simulink model "Quaternion_from_NodeMCU"  (R2018b)
settings: Solver=VariableStepAuto  StartTime=0.0  StopTime=inf  FixedStep=0.01  RelTol=1e-3
undefined symbols (not defined in the file): LF, serial
libraries: instrumentlib x4, sm_lib x4, nesl_utility x4, sharedtransform x1
settings Model: Creator=gelli  LastModifiedBy=gelli

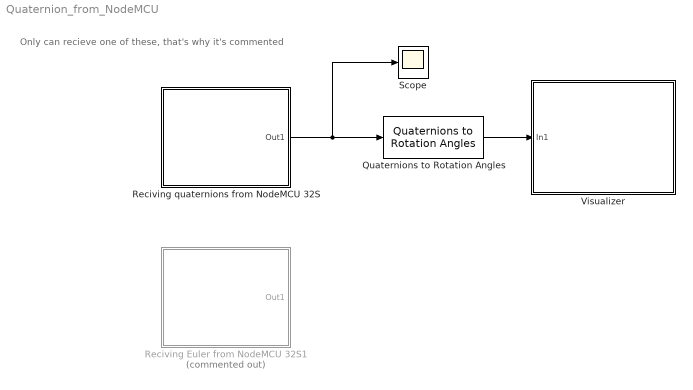
== system Quaternion_from_NodeMCU ==
  note: Only can recieve one of these, that's why it's commented
  Quaternions to Rotation Angles : sharedtransform/Quaternions to Rotation Angles  rotationOrder=XYZ  aMode=aMode
      settings: SourceProductBaseCode=AE
  Reciving Euler from NodeMCU 32S1 : Subsystem  Commented=on
      mask Display: image('Picture_of_NodeMCU.jpg');
  Reciving quaternions from NodeMCU 32S : Subsystem
      mask Display: image('Picture_of_NodeMCU.jpg');
  Scope : Scope
  Visualizer : Subsystem
  wires:
  Reciving quaternions from NodeMCU 32S/1(Out1) -> Quaternions to Rotation Angles/1, Scope/1
  Quaternions to Rotation Angles/1 -> Visualizer/1(In1)

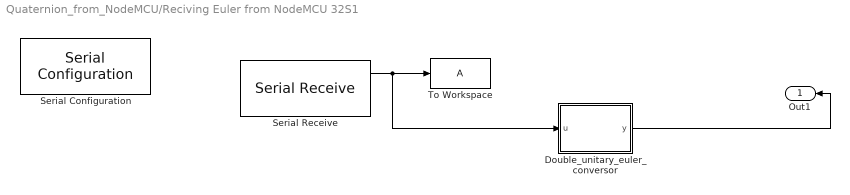
== system Quaternion_from_NodeMCU/Reciving Euler from NodeMCU 32S1 ==
  Double_unitary_euler_conversor : MATLAB Function  TreatAsAtomicUnit=on
  Serial Configuration : instrumentlib/Serial Configuration  Priority=-200000  ComPortMenu=COM6  ComPort=COM6  ObjConstructor=serial('COM6');  BaudRate=115200  DataBits=8  Parity=none  StopBits=1  FlowControl=none  Timeout=10  ByteOrder=LittleEndian
  Serial Receive : instrumentlib/Serial Receive  ComPortMenu=COM6  ComPort=COM6  ObjConstructor=serial('COM6');  Header=R  Terminator=LF ('\n')  DataSize=3  DataType=uint8  EnableBlockingMode=off  ActionDataUnavailable=Output last received value  CustomValue=0  SampleTime=0.001
  To Workspace : ToWorkspace  VariableName=A  SaveFormat=Timeseries  SampleTime=-1
  Out1 : Outport
  wires:
  Double_unitary_euler_conversor/1(y) -> Out1/1
  Serial Receive/1 -> Double_unitary_euler_conversor/1(u), To Workspace/1

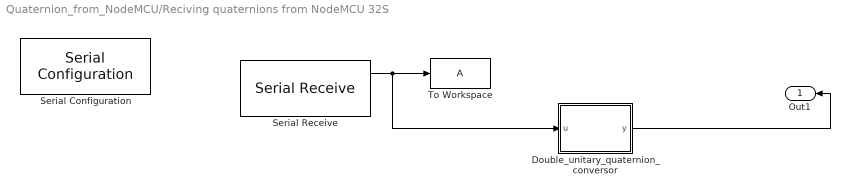
== system Quaternion_from_NodeMCU/Reciving quaternions from NodeMCU 32S ==
  Double_unitary_quaternion_conversor : MATLAB Function  TreatAsAtomicUnit=on
  Serial Configuration : instrumentlib/Serial Configuration  Priority=-200000  ComPortMenu=COM6  ComPort=COM6  ObjConstructor=serial('COM6');  BaudRate=115200  DataBits=8  Parity=none  StopBits=1  FlowControl=none  Timeout=10  ByteOrder=LittleEndian
  Serial Receive : instrumentlib/Serial Receive  ComPortMenu=COM6  ComPort=COM6  ObjConstructor=serial('COM6');  Header=R  Terminator=LF ('\n')  DataSize=4  DataType=uint8  EnableBlockingMode=off  ActionDataUnavailable=Output last received value  CustomValue=0  SampleTime=0.01
  To Workspace : ToWorkspace  VariableName=A  SaveFormat=Timeseries  SampleTime=-1
  Out1 : Outport
  wires:
  Double_unitary_quaternion_conversor/1(y) -> Out1/1
  Serial Receive/1 -> Double_unitary_quaternion_conversor/1(u), To Workspace/1

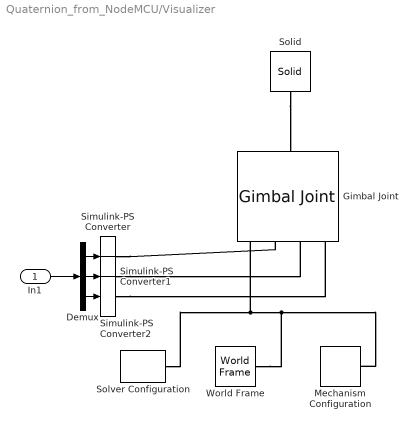
== system Quaternion_from_NodeMCU/Visualizer ==
  In1 : Inport
  Demux : Demux  Outputs=3
  Gimbal Joint : sm_lib/Joints/Gimbal Joint  SenseConstraintForce=off  SenseConstraintForceX=off  SenseConstraintForceY=off  SenseConstraintForceZ=off  SenseConstraintTorque=off  SenseConstraintTorqueX=off  SenseConstraintTorqueY=off  SenseConstraintTorqueZ=off  SenseTotalForce=off  SenseTotalForceX=off  SenseTotalForceY=off  SenseTotalForceZ=off  SenseTotalTorque=off  SenseTotalTorqueX=off  SenseTotalTorqueY=off  SenseTotalTorqueZ=off  CompositeWrenchDir=FollowerOnBase  CompositeWrenchFrame=BaseFrame  RxEquilibriumPosition=0  RxEquilibriumPositionUnits=deg  RxSpringStiffness=0  RxSpringStiffnessUnits=N*m/deg  RxDampingCoefficient=0  RxDampingCoefficientUnits=N*m/(deg/s)  RxTorqueActuationMode=ComputedTorque  RxMotionActuationMode=InputMotion  RxSensePosition=off  RxSenseVelocity=off  RxSenseAcceleration=off  RxSenseTorqueForce=off  RxPositionTargetSpecify=off  RxPositionTargetPriority=High  RxPositionTargetValue=0  RxPositionTargetValueUnits=deg  RxVelocityTargetSpecify=off  RxVelocityTargetPriority=High  RxVelocityTargetValue=0  RxVelocityTargetValueUnits=deg/s  RyEquilibriumPosition=0  RyEquilibriumPositionUnits=deg  RySpringStiffness=0  RySpringStiffnessUnits=N*m/deg  RyDampingCoefficient=0  RyDampingCoefficientUnits=N*m/(deg/s)  RyTorqueActuationMode=ComputedTorque  RyMotionActuationMode=InputMotion  RySensePosition=off  RySenseVelocity=off  RySenseAcceleration=off  RySenseTorqueForce=off  RyPositionTargetSpecify=off  RyPositionTargetPriority=High  RyPositionTargetValue=0  RyPositionTargetValueUnits=deg  RyVelocityTargetSpecify=off  RyVelocityTargetPriority=High  RyVelocityTargetValue=0  RyVelocityTargetValueUnits=deg/s  RzEquilibriumPosition=0  RzEquilibriumPositionUnits=deg  RzSpringStiffness=0  RzSpringStiffnessUnits=N*m/deg  RzDampingCoefficient=0  RzDampingCoefficientUnits=N*m/(deg/s)  RzTorqueActuationMode=ComputedTorque  RzMotionActuationMode=InputMotion  RzSensePosition=off  RzSenseVelocity=off  RzSenseAcceleration=off  RzSenseTorqueForce=off  RzPositionTargetSpecify=off  RzPositionTargetPriority=High  RzPositionTargetValue=0  RzPositionTargetValueUnits=deg  RzVelocityTargetSpecify=off  RzVelocityTargetPriority=High  RzVelocityTargetValue=0  RzVelocityTargetValueUnits=deg/s
      settings: SourceProductName=Simscape Multibody
  Mechanism Configuration : sm_lib/Utilities/Mechanism Configuration  UniformGravity=Constant  GravityVector=[0 0 -9.80665]  GravityUnits=m/s^2  LinearizationDelta=0.001
  Simulink-PS Converter : nesl_utility/Simulink-PS Converter  PhysicalDomain=network_engine_domain  SubClassName=ps_input  LeftPortType=input  RightPortType=output  PseudoPeriodic=off  Frequencies=[]  NoiseDistribution=none  NoiseParameters=[]  Unit=1  AffineConversion=off  FilteringAndDerivatives=zero  SimscapeFilterOrder=1  InputFilterTimeConstant=0.01  UdotUserProvided=1
  Simulink-PS Converter1 : nesl_utility/Simulink-PS Converter  PhysicalDomain=network_engine_domain  SubClassName=ps_input  LeftPortType=input  RightPortType=output  PseudoPeriodic=off  Frequencies=[]  NoiseDistribution=none  NoiseParameters=[]  Unit=1  AffineConversion=off  FilteringAndDerivatives=zero  SimscapeFilterOrder=1  InputFilterTimeConstant=0.01  UdotUserProvided=1
  Simulink-PS Converter2 : nesl_utility/Simulink-PS Converter  PhysicalDomain=network_engine_domain  SubClassName=ps_input  LeftPortType=input  RightPortType=output  PseudoPeriodic=off  Frequencies=[]  NoiseDistribution=none  NoiseParameters=[]  Unit=1  AffineConversion=off  FilteringAndDerivatives=zero  SimscapeFilterOrder=1  InputFilterTimeConstant=0.01  UdotUserProvided=1
  Solid : sm_lib/Body Elements/Solid  InertiaType=CalculateFromGeometry  Mass=1  MassUnits=kg  CenterOfMass=[0 0 0]  CenterOfMassUnits=m  MomentsOfInertia=[1 1 1]  MomentsOfInertiaUnits=kg*m^2  ProductsOfInertia=[0 0 0]  ProductsOfInertiaUnits=kg*m^2  BasedOnType=Density  Density=1000  DensityUnits=kg/m^3  DoExposeReferenceFrame=on  SerializedFrames=<Frames/>  GraphicType=FromGeometry  MarkerShape=Sphere  MarkerSize=10  GraphicVisPropType=SimpleVisualProperties  GraphicDiffuseColor=[1.0 0.4 0.2]  GraphicSpecularColor=[0.5 0.5 0.5 1.0]  GraphicAmbientColor=[0.15 0.15 0.15 1.0]  GraphicEmissiveColor=[0.0 0.0 0.0 1.0]  GraphicShininess=75  GraphicOpacity=1.0  GeometryShape=Brick  RectangleSize=[1 1]  RectangleSizeUnits=m  BrickDimensions=[1 1 1]  BrickDimensionUnits=m  CylinderRadius=1  CylinderRadiusUnits=m  CylinderLength=1  CylinderLengthUnits=m  SphereRadius=1  SphereRadiusUnits=m  EllipsoidRadii=[1 1 1]  EllipsoidRadiiUnits=m  ExtrusionCrossSection=[1 1; -1 1; -1 -1; 1 -1]  ExtrusionCrossSectionUnits=m  ExtrusionLength=1  ExtrusionLengthUnits=m  PolygonNumSides=3  PolygonOuterRadius=1  PolygonOuterRadiusUnits=m  ExtGeomFileType=STEP  ExtGeomFileUnits=m  RevolutionCrossSection=[1 1; 1 -1; 2 -1; 2 1]  RevolutionCrossSectionUnits=m  RevolutionExtent=Full  RevolutionAngle=180  RevolutionAngleUnits=deg
  Solver Configuration : nesl_utility/Solver Configuration  PhysicalDomain=network_engine_domain  SubClassName=solver  LeftPortType=input  RightPortType=generic  Tones=[]  Harmonics=[]  SimulateNoise=off  Profile=off  UseLocalSampling=off  EnableSwitchedLinearOptims=on  FrequencyDomain=off  UseCCode=off  RelTol=0.001  AbsTol=1e-06  MinStep=1e-09  ToWorkspace=off  RevertToSquareIcSolve=off  NumHomotopyIterations=100  PhasorMode=off  PhasorModeNumHarmonics=1  DoDC=off  ResidualTolerance=1e-09  UseLocalSolver=off  LocalSolverChoice=NE_BACKWARD_EULER_ADVANCER  LocalSolverSampleTime=0.001  DoFixedCost=off  MaxNonlinIter=3  MaxModeIter=2  LinearAlgebra=auto  EquationFormulation=NE_TIME_EF  DelaysMemoryBudget=1024  AutomaticFiltering=on  FilteringTimeConstant=0.001  PartitionStorageMethod=AS_NEEDED  PartitionMemoryBudget=1024
  World Frame : sm_lib/Frames and Transforms/World Frame
  wires:
  In1/1 -> Demux/1
  Demux/1 -> Simulink-PS Converter/1
  Demux/2 -> Simulink-PS Converter1/1
  Demux/3 -> Simulink-PS Converter2/1
  connections:
  Solver Configuration/RConn1 -- Mechanism Configuration/RConn1 -- World Frame/RConn1 -- Gimbal Joint/LConn1
  Solid/RConn1 -- Gimbal Joint/RConn1
  Simulink-PS Converter/RConn1 -- Gimbal Joint/LConn2
  Simulink-PS Converter1/RConn1 -- Gimbal Joint/LConn3
  Simulink-PS Converter2/RConn1 -- Gimbal Joint/LConn4

== matlab function Quaternion_from_NodeMCU/Reciving Euler from NodeMCU 32S1/Double_unitary_euler_conversor ==
  data: u input; y output
function y = fcn(u)

y = (360*double(u)/255)-180 ;

y = y*pi/180; % Conversion to radians

== matlab function Quaternion_from_NodeMCU/Reciving quaternions from NodeMCU 32S/Double_unitary_quaternion_conversor ==
  data: u input; y output
function y = fcn(u)

y = (double(u)-127)/127 ;
